simulink model "pid_signal"  (R2021b)
settings: Solver=VariableStepAuto  StartTime=0.0  StopTime=10.0  RelTol=1e-3
values from neighbouring files (symbols this model uses):
  D_Max = Simulink.Parameter    [pid_signal.m]
  D_Min = Simulink.Parameter    [pid_signal.m]
  I_Max = Simulink.Parameter    [pid_signal.m]
  I_Min = Simulink.Parameter    [pid_signal.m]
  Kd = Simulink.Parameter    [pid_signal.m]
  Ki = Simulink.Parameter    [pid_signal.m]
  Kp = Simulink.Parameter    [pid_signal.m]
  Sample_Time = Simulink.Parameter    [pid_signal.m]
undefined symbols (not defined in the file or in its folder): Out_Max, Out_Min
libraries: simulink x3
settings Model: Creator=youth_zhao_58169  LastModifiedBy=youth_zhao_58169

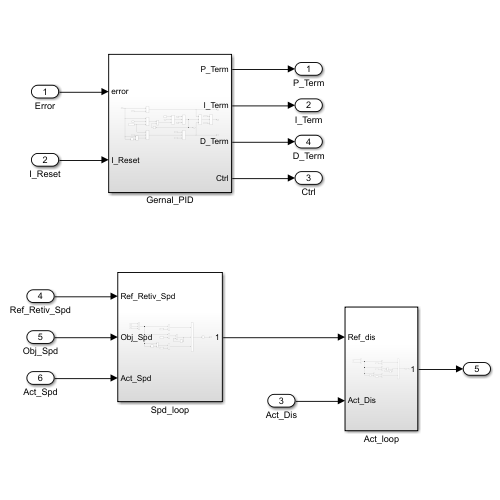
[thumbnail: Simulink's stored preview of the top-level diagram]
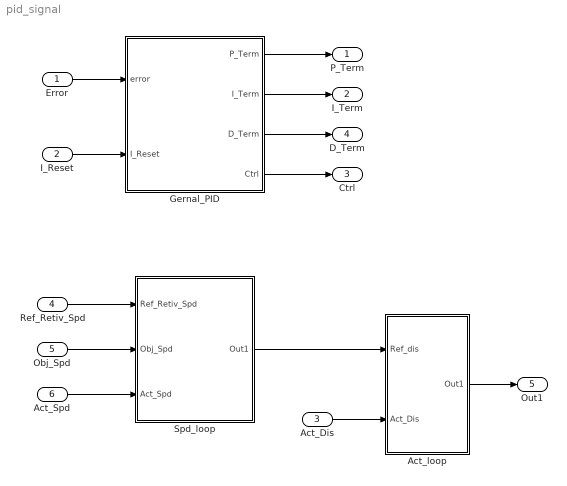
== system pid_signal ==
  Error : Inport
  I_Reset : Inport  Port=2
  Act_Dis : Inport  Port=3
  Ref_Retiv_Spd : Inport  Port=4
  Obj_Spd : Inport  Port=5
  Act_Spd : Inport  Port=6
  Act_loop : Subsystem
  Gernal_PID : Subsystem
  Spd_loop : Subsystem
  P_Term : Outport
  I_Term : Outport  Port=2
  Ctrl : Outport  Port=3
  D_Term : Outport  Port=4
  Out1 : Outport  Port=5
  wires:
  Error/1 -> Gernal_PID/1(error)
  I_Reset/1 -> Gernal_PID/2(I_Reset)
  Gernal_PID/1(P_Term) -> P_Term/1
  Gernal_PID/2(I_Term) -> I_Term/1
  Gernal_PID/4(Ctrl) -> Ctrl/1
  Gernal_PID/3(D_Term) -> D_Term/1
  Spd_loop/1(Out1) -> Act_loop/1(Ref_dis)
  Act_Dis/1 -> Act_loop/2(Act_Dis)
  Act_loop/1(Out1) -> Out1/1
  Ref_Retiv_Spd/1 -> Spd_loop/1(Ref_Retiv_Spd)
  Obj_Spd/1 -> Spd_loop/2(Obj_Spd)
  Act_Spd/1 -> Spd_loop/3(Act_Spd)

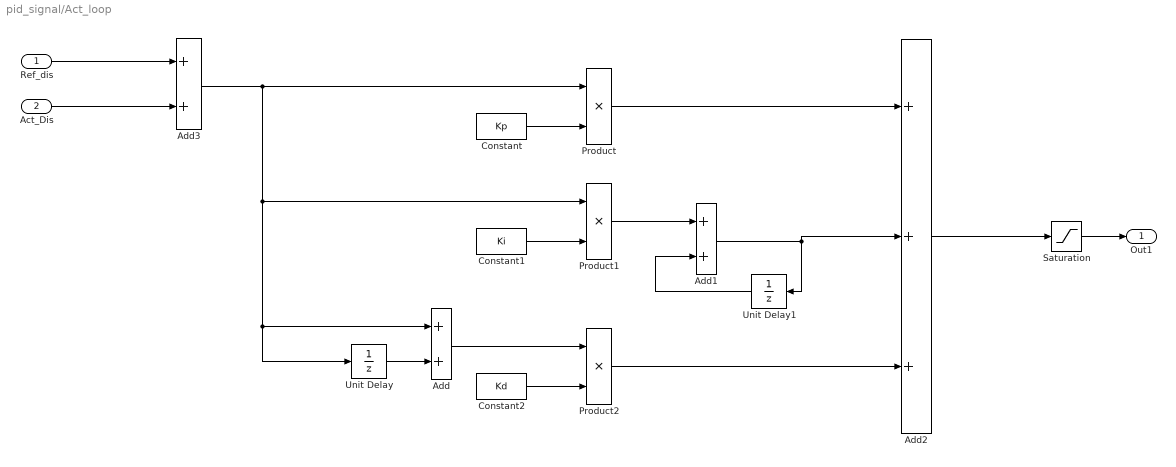
== system pid_signal/Act_loop ==
  Ref_dis : Inport
  Act_Dis : Inport  Port=2
  Add : Sum
  Add1 : Sum
  Add2 : Sum  Inputs=+++
  Add3 : Sum
  Constant : Constant  Value=Kp
  Constant1 : Constant  Value=Ki
  Constant2 : Constant  Value=Kd
  Product : Product
  Product1 : Product
  Product2 : Product
  Saturation : Saturate
  Unit Delay : UnitDelay  SampleTime=-1  HasFrameUpgradeWarning=on
  Unit Delay1 : UnitDelay  SampleTime=-1  HasFrameUpgradeWarning=on
  Out1 : Outport
  wires:
  Add3/1 -> Product1/1, Add/1, Unit Delay/1, Product/1
  Add1/1 -> Add2/2, Unit Delay1/1
  Ref_dis/1 -> Add3/1
  Product/1 -> Add2/1
  Product2/1 -> Add2/3
  Add/1 -> Product2/1
  Add2/1 -> Saturation/1
  Unit Delay/1 -> Add/2
  Product1/1 -> Add1/1
  Unit Delay1/1 -> Add1/2
  Constant1/1 -> Product1/2
  Constant2/1 -> Product2/2
  Constant/1 -> Product/2
  Act_Dis/1 -> Add3/2
  Saturation/1 -> Out1/1

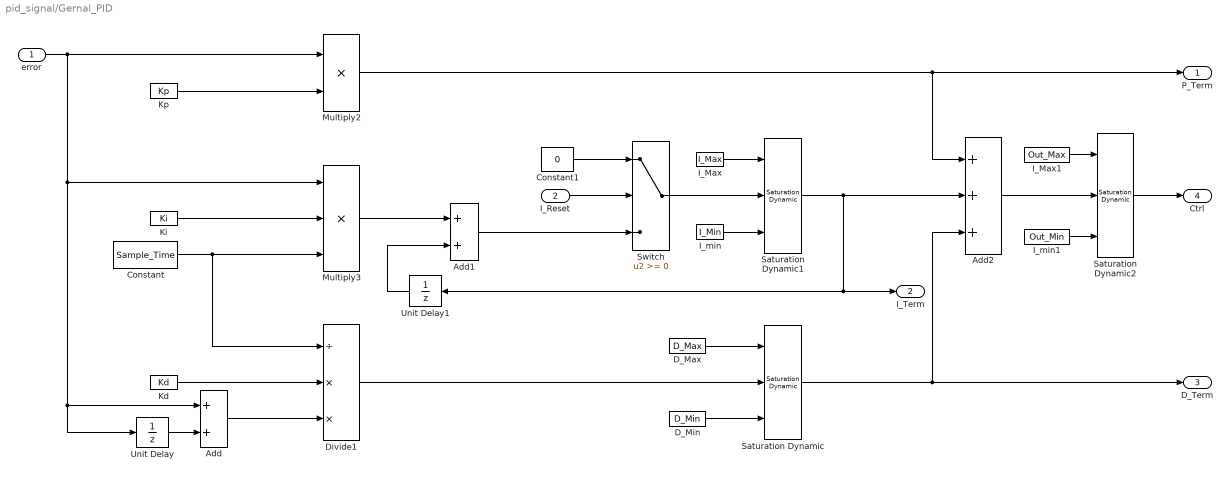
== system pid_signal/Gernal_PID ==
  error : Inport
  I_Reset : Inport  Port=2
  Add : Sum
  Add1 : Sum
  Add2 : Sum  Inputs=+++
  Constant : Constant  Value=Sample_Time
  Constant1 : Constant  Value=0  VectorParams1D=off  OutDataTypeStr=single
  D_Max : Constant  Value=D_Max
  D_Min : Constant  Value=D_Min
  Divide1 : Product  Inputs=/**
  I_Max : Constant  Value=I_Max
  I_Max1 : Constant  Value=Out_Max
  I_min : Constant  Value=I_Min
  I_min1 : Constant  Value=Out_Min
  Kd : Constant  Value=Kd
  Ki : Constant  Value=Ki
  Kp : Constant  Value=Kp
  Multiply2 : Product
  Multiply3 : Product  Inputs=3
  Saturation Dynamic : simulink/Discontinuities/Saturation Dynamic  OutMin=[]  OutMax=[]  OutDataTypeStr=Inherit: Same as second input  OutDataType=fixdt(1, 16)  OutScaling=2^-10  DoSatur=off
  Saturation Dynamic1 : simulink/Discontinuities/Saturation Dynamic  OutMin=[]  OutMax=[]  OutDataTypeStr=Inherit: Same as second input  OutDataType=fixdt(1, 16)  OutScaling=2^-10  DoSatur=off
  Saturation Dynamic2 : simulink/Discontinuities/Saturation Dynamic  OutMin=[]  OutMax=[]  OutDataTypeStr=Inherit: Same as second input  OutDataType=fixdt(1, 16)  OutScaling=2^-10  DoSatur=off
  Switch : Switch  OutDataTypeStr=Inherit: Inherit via back propagation
  Unit Delay : UnitDelay  SampleTime=-1  StateName=I_Term_Last  HasFrameUpgradeWarning=on
  Unit Delay1 : UnitDelay  SampleTime=-1  StateName=Err_Last  HasFrameUpgradeWarning=on
  P_Term : Outport
  I_Term : Outport  Port=2
  D_Term : Outport  Port=3
  Ctrl : Outport  Port=4
  wires:
  Constant1/1 -> Switch/1
  Saturation Dynamic1/1 -> Add2/2, I_Term/1, Unit Delay1/1
  Ki/1 -> Multiply3/2
  Unit Delay1/1 -> Add1/2
  D_Min/1 -> Saturation Dynamic/3
  I_Max/1 -> Saturation Dynamic1/1
  Saturation Dynamic/1 -> D_Term/1, Add2/3
  Kp/1 -> Multiply2/2
  Add2/1 -> Saturation Dynamic2/2
  Multiply2/1 -> P_Term/1, Add2/1
  Add/1 -> Divide1/3
  Kd/1 -> Divide1/2
  Add1/1 -> Switch/3
  error/1 -> Multiply3/1, Unit Delay/1, Add/1, Multiply2/1
  Divide1/1 -> Saturation Dynamic/2
  D_Max/1 -> Saturation Dynamic/1
  Switch/1 -> Saturation Dynamic1/2
  Multiply3/1 -> Add1/1
  I_Reset/1 -> Switch/2
  Constant/1 -> Divide1/1, Multiply3/3
  I_min/1 -> Saturation Dynamic1/3
  Unit Delay/1 -> Add/2
  I_Max1/1 -> Saturation Dynamic2/1
  I_min1/1 -> Saturation Dynamic2/3
  Saturation Dynamic2/1 -> Ctrl/1

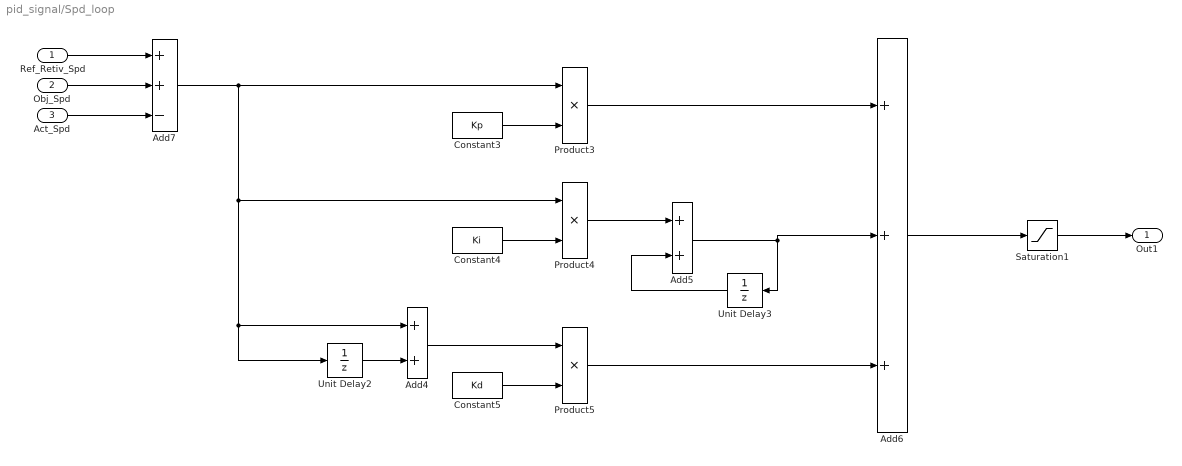
== system pid_signal/Spd_loop ==
  Ref_Retiv_Spd : Inport
  Obj_Spd : Inport  Port=2
  Act_Spd : Inport  Port=3
  Add4 : Sum
  Add5 : Sum
  Add6 : Sum  Inputs=+++
  Add7 : Sum  Inputs=++-
  Constant3 : Constant  Value=Kp
  Constant4 : Constant  Value=Ki
  Constant5 : Constant  Value=Kd
  Product3 : Product
  Product4 : Product
  Product5 : Product
  Saturation1 : Saturate
  Unit Delay2 : UnitDelay  SampleTime=-1  HasFrameUpgradeWarning=on
  Unit Delay3 : UnitDelay  SampleTime=-1  HasFrameUpgradeWarning=on
  Out1 : Outport
  wires:
  Constant3/1 -> Product3/2
  Unit Delay3/1 -> Add5/2
  Constant5/1 -> Product5/2
  Obj_Spd/1 -> Add7/2
  Constant4/1 -> Product4/2
  Add5/1 -> Add6/2, Unit Delay3/1
  Add7/1 -> Product4/1, Add4/1, Unit Delay2/1, Product3/1
  Saturation1/1 -> Out1/1
  Product3/1 -> Add6/1
  Product4/1 -> Add5/1
  Unit Delay2/1 -> Add4/2
  Product5/1 -> Add6/3
  Add6/1 -> Saturation1/1
  Add4/1 -> Product5/1
  Act_Spd/1 -> Add7/3
  Ref_Retiv_Spd/1 -> Add7/1
